simulink model "testnrlmsise00_model"  (R2024a)
settings: Solver=FixedStepDiscrete  StartTime=0.0  StopTime=1  FixedStep=1  RelTol=1e-3
settings Model: PauseTimes=47  Creator=Friedrich Tuttas  LastModifiedBy=Friedrich Tuttas
settings RTWCC: GPUComputeCapability=3.5

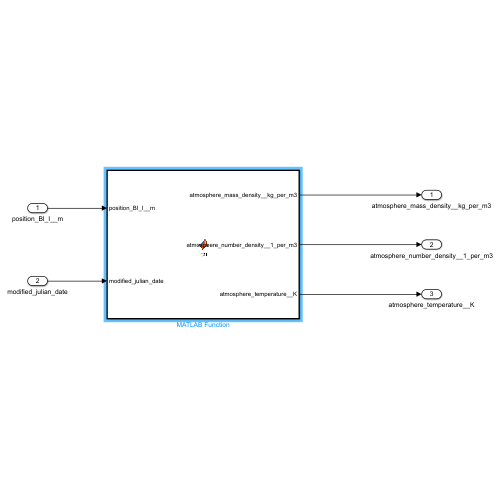
[thumbnail: Simulink's stored preview of the top-level diagram]
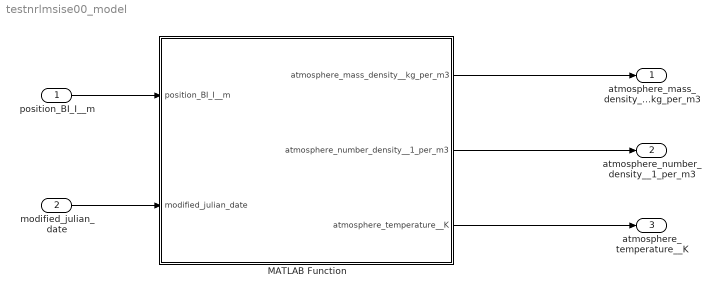
== system testnrlmsise00_model ==
  position_BI_I__m : Inport  PortDimensions=[3,1]
  modified_julian_date : Inport  Port=2
  MATLAB Function : MATLAB Function  TreatAsAtomicUnit=on
  atmosphere_mass_density__kg_per_m3 : Outport
  atmosphere_number_density__1_per_m3 : Outport  Port=2
  atmosphere_temperature__K : Outport  Port=3
  wires:
  MATLAB Function/1(atmosphere_mass_density__kg_per_m3) -> atmosphere_mass_density__kg_per_m3/1
  position_BI_I__m/1 -> MATLAB Function/1(position_BI_I__m)
  modified_julian_date/1 -> MATLAB Function/2(modified_julian_date)
  MATLAB Function/2(atmosphere_number_density__1_per_m3) -> atmosphere_number_density__1_per_m3/1
  MATLAB Function/3(atmosphere_temperature__K) -> atmosphere_temperature__K/1

== matlab function testnrlmsise00_model/MATLAB Function ==
  data: position_BI_I__m input; atmosphere_mass_density__kg_per_m3 output; modified_julian_date input; atmosphere_number_density__1_per_m3 output; atmosphere_temperature__K output; Parameters parameter
function [atmosphere_mass_density__kg_per_m3, atmosphere_number_density__1_per_m3, atmosphere_temperature__K] = fcn(position_BI_I__m, modified_julian_date, Parameters)


[atmosphere_mass_density__kg_per_m3, atmosphere_number_density__1_per_m3, atmosphere_temperature__K] = Nrlmsise00.execute(position_BI_I__m, [1; 0; 0; 0], modified_julian_date, Parameters);
